simulink model "subsytem_masking"  (R2015b)
settings: Solver=FixedStepDiscrete  StartTime=0.0  StopTime=Inf  RelTol=1e-3
settings Model: Creator=Shravankumar147  LastModifiedBy=Shravankumar147

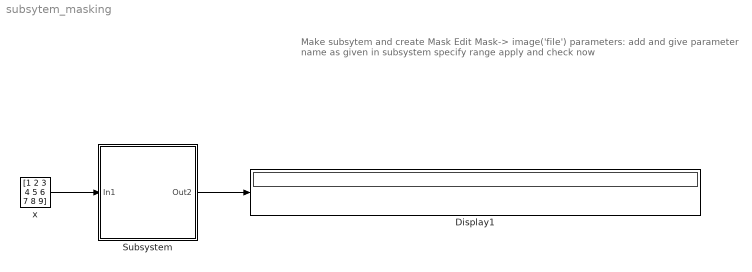
== system subsytem_masking ==
  note: Make subsytem and create Mask
      | Edit Mask-> image('file')
      | parameters: add and give parameter name as given in subsystem
      | specify range
      | apply and check now
  Display1 : Display
  Subsystem : Subsystem  mask{c=1, m=64.0}
      mask prompts: c "const"; m "slope"
      mask TypeOptions c: 1 | 2 | 3 | 4
      mask Display: image('D:\Educational\MATLAB\proj_expo\Tutorial\coursera.png')
  x : Constant  Value=[1 2 3 4 5 6 7 8 9]
  wires:
  Subsystem/1(Out2) -> Display1/1
  x/1 -> Subsystem/1(In1)

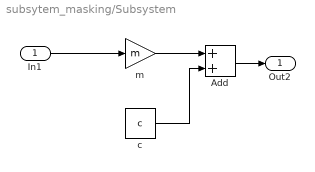
== system subsytem_masking/Subsystem ==
  In1 : Inport
  Add : Sum
  c : Constant  Value=c
  m : Gain  Gain=m
  Out2 : Outport
  wires:
  In1/1 -> m/1
  Add/1 -> Out2/1
  m/1 -> Add/1
  c/1 -> Add/2
